simulink model "multiModePlanner"  (R2020b)
settings: Solver=FixedStepAuto  StartTime=0.0  StopTime=inf  FixedStep=0.5  MinStep=0.1  RelTol=1e-3
undefined symbols (not defined in the file or in its folder): DiscIntNeverNeededParam
settings Model: Creator=Ron  LastModifiedBy=cosorio
settings DataIOCC: ReturnWorkspaceOutputs=off

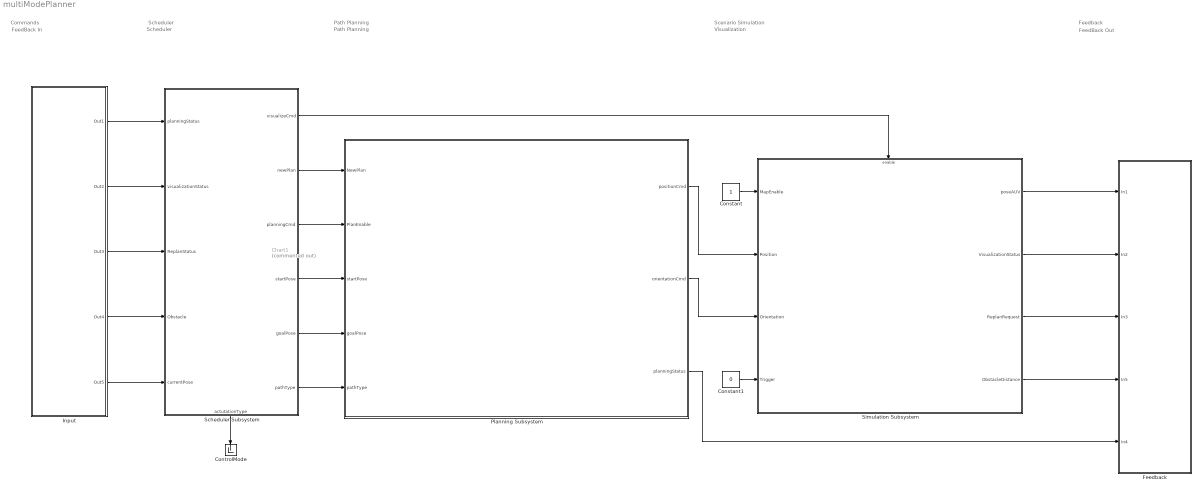
== system multiModePlanner ==
  note: Path Planning
  note: FeedBack In
  note: FeedBack Out
  note: Scheduler
  note: Path Planning
  note: Visualization
  note: Scheduler
  note: Commands
  note: Feedback
  note: Scenario Simulation
  " Feedback  " : Subsystem
  Chart1 : Stateflow chart  Commented=on  TreatAsAtomicUnit=on
  Constant : Constant
  Constant1 : Constant  Value=0
  ControlMode : Terminator
  Input : Subsystem
  Planning Subsystem : Subsystem
  Scheduler Subsystem : Stateflow chart  TreatAsAtomicUnit=on
      settings: PortSchema="{\"entries\":[{\"content\":{\"sides\":[{\"content\":{\"connectorIds\":[\"In1\",\"In2\",\"In3\",\"In4\",\"In5\"]},\"type\":\"ConnectorPlacement.EquallySpacedRectSide\",\"uuid\":\"1bd6ddfe-5f8a-4931-8a8b-c6c0dc399580\"},{\"content\":{\"connectorIds\":[\"Out5\",\"Out6\",\"Out1\",\"Out2\",\"Out3\",\"Out4\"],\"side\":\"RIGHT\"},\"type\":\"ConnectorPlacement.EquallySpacedRectSide\",\"uuid\":\"6c4632f4-be38-4d28-9a15-6462af5cd566\"},{\"content\":{\"connectorIds\":[],\"side\":\"TOP\"},\"type\":\"ConnectorPlacement.EquallySpacedRectSide\",\"uuid\":\"b3d6ad09-cf01-4725-a10c-99a606f09fed\"},{\"content\":{\"connectorIds\":[\"Out7\"],\"side\":\"BOTTOM\"},\"type\":\"ConnectorPlacement.EquallySpacedRectSide\",\"uuid\":\"99f6d769-50a8-4e4e-9c90-fdb41bcec8c1\"}]},\"type\":\"ConnectorPlacement.EquallySpacedConnector\",\"uuid\":\"51f2bfa3-614b-4c29-a9f7-1bf781273fcd\"}],\"packageUris\":[\"http://schema.mathworks.com/mf0/Connector/19700101\"],\"version\":\"1.0\"}"
  Simulation Subsystem : Subsystem
  wires:
  Constant/1 -> Simulation Subsystem/1(MapEnable)
  Constant1/1 -> Simulation Subsystem/4(Trigger)
  Scheduler Subsystem/5(visualizeCmd) -> Simulation Subsystem/Enable
  Scheduler Subsystem/7(actutationType) -> ControlMode/1
  Scheduler Subsystem/6(newPlan) -> Planning Subsystem/1(NewPlan)
  Scheduler Subsystem/1(planningCmd) -> Planning Subsystem/2(" PlanEnable")
  Scheduler Subsystem/2(startPose) -> Planning Subsystem/3(startPose)
  Scheduler Subsystem/3(goalPose) -> Planning Subsystem/4(goalPose)
  Scheduler Subsystem/4(pathType) -> Planning Subsystem/5(pathType)
  Planning Subsystem/1(positionCmd) -> Simulation Subsystem/2(Position)
  Planning Subsystem/2(orientationCmd) -> Simulation Subsystem/3(Orientation)
  Input/1(Out1) -> Scheduler Subsystem/1(planningStatus)
  Input/2(Out2) -> Scheduler Subsystem/2(visualizationStatus)
  Input/3(Out3) -> Scheduler Subsystem/3(ReplanStatus)
  Input/4(Out4) -> Scheduler Subsystem/4(Obstacle)
  Input/5(Out5) -> Scheduler Subsystem/5(currentPose)
  Simulation Subsystem/1(poseAUV) -> " Feedback  "/1(In1)
  Simulation Subsystem/2(VisualizationStatus) -> " Feedback  "/2(In2)
  Simulation Subsystem/3(ReplanRequest) -> " Feedback  "/3(In3)
  Planning Subsystem/3(planningStatus) -> " Feedback  "/5(In4)
  Simulation Subsystem/4(ObstacleDistance) -> " Feedback  "/4(In5)

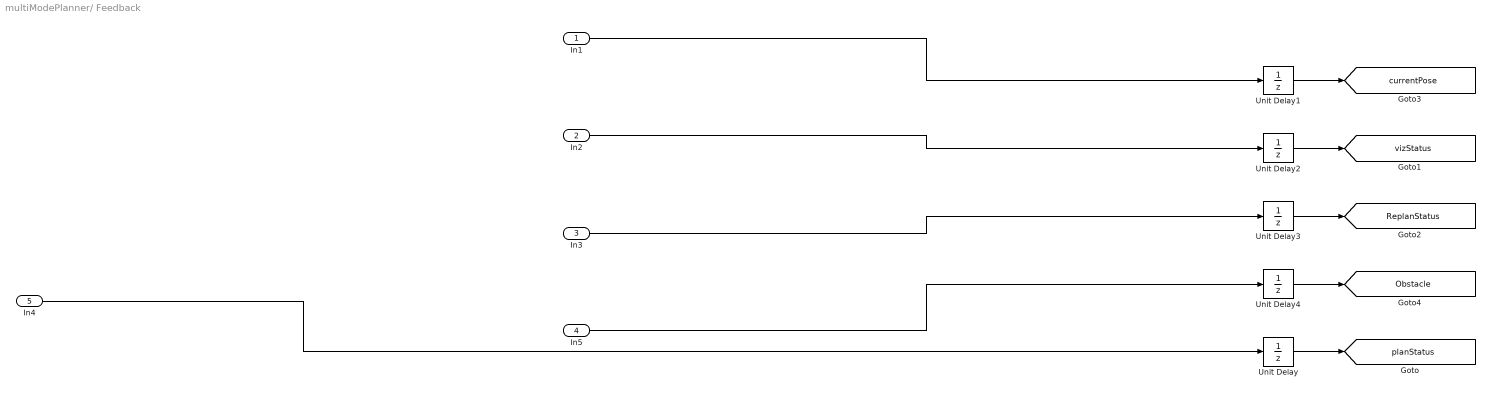
== system multiModePlanner/ Feedback   ==
  In1 : Inport
  In2 : Inport  Port=2
  In3 : Inport  Port=3
  In5 : Inport  Port=4
  In4 : Inport  Port=5
  Unit Delay{,1..3} (4 alike) : UnitDelay  SampleTime=-1  HasFrameUpgradeWarning=on
  Unit Delay4 : UnitDelay  InitialCondition=[0]  SampleTime=-1  HasFrameUpgradeWarning=on
  tag scope: Obstacle=global, ReplanStatus=global, currentPose=global, planStatus=global, vizStatus=global
  wires:
  Unit Delay3/1 -> [ReplanStatus]
  In2/1 -> Unit Delay2/1
  Unit Delay1/1 -> [currentPose]
  Unit Delay/1 -> [planStatus]
  In3/1 -> Unit Delay3/1
  Unit Delay4/1 -> [Obstacle]
  Unit Delay2/1 -> [vizStatus]
  In1/1 -> Unit Delay1/1
  In5/1 -> Unit Delay4/1
  In4/1 -> Unit Delay/1

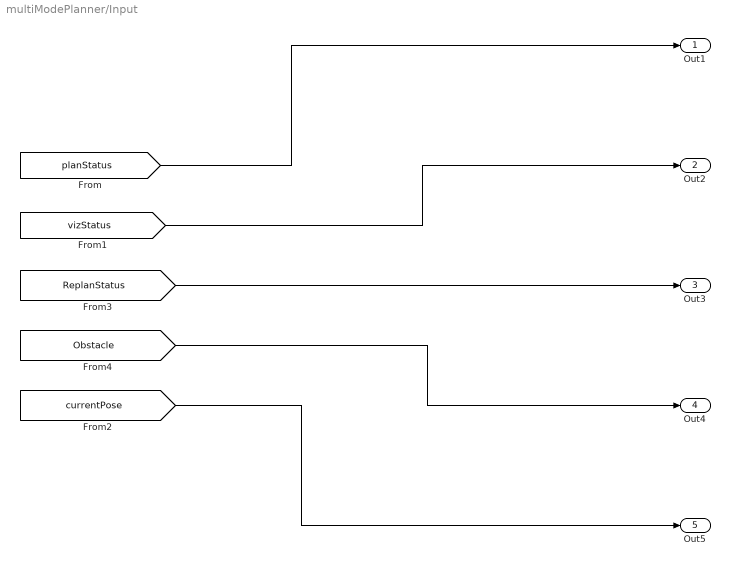
== system multiModePlanner/Input ==
  Out1 : Outport
  Out2 : Outport  Port=2
  Out3 : Outport  Port=3
  Out4 : Outport  Port=4
  Out5 : Outport  Port=5
  wires:
  [vizStatus] -> Out2/1
  [ReplanStatus] -> Out3/1
  [planStatus] -> Out1/1
  [currentPose] -> Out5/1
  [Obstacle] -> Out4/1

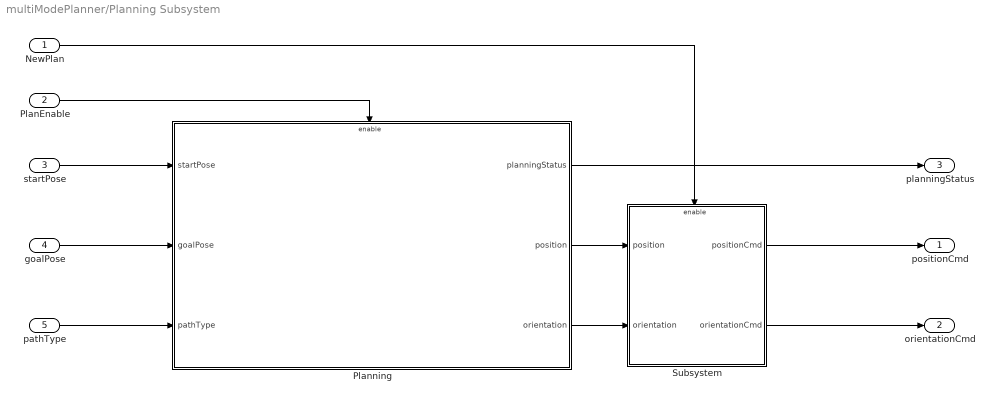
== system multiModePlanner/Planning Subsystem ==
  NewPlan : Inport
  " PlanEnable" : Inport  Port=2
  startPose : Inport  Port=3
  goalPose : Inport  Port=4
  pathType : Inport  Port=5
  Planning : Subsystem
  Subsystem : Subsystem
  positionCmd : Outport
  orientationCmd : Outport  Port=2
  planningStatus : Outport  Port=3
  wires:
  Planning/1(planningStatus) -> planningStatus/1
  Planning/3(orientation) -> Subsystem/2(orientation)
  pathType/1 -> Planning/3(pathType)
  Planning/2(position) -> Subsystem/1(position)
  Subsystem/1(positionCmd) -> positionCmd/1
  startPose/1 -> Planning/1(startPose)
  Subsystem/2(orientationCmd) -> orientationCmd/1
  " PlanEnable"/1 -> Planning/Enable
  goalPose/1 -> Planning/2(goalPose)
  NewPlan/1 -> Subsystem/Enable

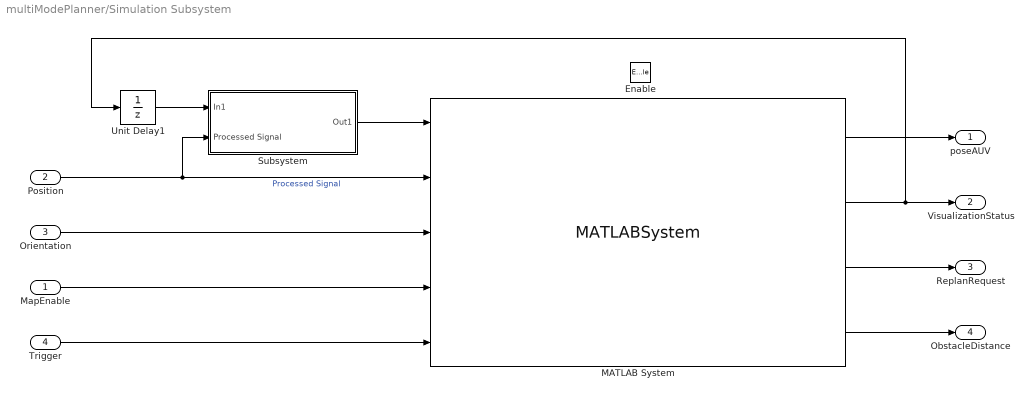
== system multiModePlanner/Simulation Subsystem ==
  MapEnable : Inport
  Position : Inport  Port=2
  Orientation : Inport  Port=3
  Trigger : Inport  Port=4
  Enable : EnablePort  PropagateVarSize=During execution
  MATLAB System : MATLABSystem  System=auvScenarioHillsSimulation_MultiMode  RollAccuracy=0.2  PitchAccuracy=0.2  YawAccuracy=0.2  PositionAccuracy=1  VelocityAccuracy=0.05
      mask Type: auvScenarioHillsSimulation_MultiMode
      mask Display:
      | disp('auvScenarioHillsSimulation_MultiMode');
      | port_label('input',1,'counter');
      | port_label('input',2,'position');
      | port_label('input',3,'orientation');
      | port_label('input',4,'mapEnable');
      | port_label('input',5,'trigger');
      | port_label('output',1,'poseUUV');
      | port_label('output',2,'VisualizationStatus');
      | port_label('output',3,'ReplanRequest');
      | port_label('output',4,'Obstacle');
  Subsystem : Subsystem
  Unit Delay1 : UnitDelay  SampleTime=-1  HasFrameUpgradeWarning=on
  poseAUV : Outport
  VisualizationStatus : Outport  Port=2
  ReplanRequest : Outport  Port=3
  ObstacleDistance : Outport  Port=4
  wires:
  Orientation/1 -> MATLAB System/3
  Trigger/1 -> MATLAB System/5
  MapEnable/1 -> MATLAB System/4
  MATLAB System/1 -> poseAUV/1
  MATLAB System/2 -> Unit Delay1/1, VisualizationStatus/1
  MATLAB System/3 -> ReplanRequest/1
  MATLAB System/4 -> ObstacleDistance/1
  Position/1 -> Subsystem/2(Processed Signal), MATLAB System/2  "Processed Signal"
  Unit Delay1/1 -> Subsystem/1(In1)
  Subsystem/1(Out1) -> MATLAB System/1

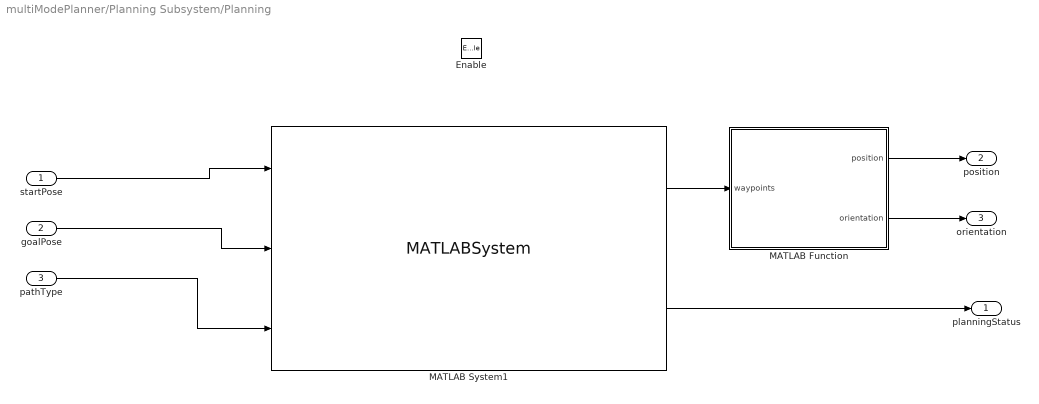
== system multiModePlanner/Planning Subsystem/Planning ==
  startPose : Inport
  goalPose : Inport  Port=2
  pathType : Inport  Port=3
  Enable : EnablePort  PropagateVarSize=During execution
  MATLAB Function : MATLAB Function  TreatAsAtomicUnit=on
  MATLAB System1 : MATLABSystem  System=auvPathPlanner_MultiMode  occMap=UUVSceneLowResMap3.mat  maxRollAngle=pi/6  airSpeed=8  flightPathAngleLimit=[ -0.1, 0.1 ]  bounds=[ -250, 250; -250, 250; -250, 250; -pi, pi ]  searchCoordinates=[ 400, 400 ]  searchFOV=10  bouyPostions=[ -150, 150, -150, -150, 150, 0 ]  bouyCoverage=300  SimulateUsing=Interpreted execution
      mask Type: auvPathPlanner_MultiMode
      mask Display:
      | disp('auvPathPlanner_MultiMode');
      | port_label('input',1,'startPose');
      | port_label('input',2,'goalPose');
      | port_label('input',3,'pathType');
      | port_label('output',1,'waypoints');
      | port_label('output',2,'planningStatus');
  planningStatus : Outport
  position : Outport  Port=2
  orientation : Outport  Port=3
  wires:
  MATLAB System1/1 -> MATLAB Function/1(waypoints)
  pathType/1 -> MATLAB System1/3
  goalPose/1 -> MATLAB System1/2
  MATLAB System1/2 -> planningStatus/1
  startPose/1 -> MATLAB System1/1
  MATLAB Function/1(position) -> position/1
  MATLAB Function/2(orientation) -> orientation/1

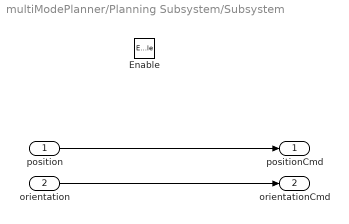
== system multiModePlanner/Planning Subsystem/Subsystem ==
  position : Inport
  orientation : Inport  Port=2
  Enable : EnablePort
  positionCmd : Outport
  orientationCmd : Outport  Port=2
  wires:
  position/1 -> positionCmd/1
  orientation/1 -> orientationCmd/1

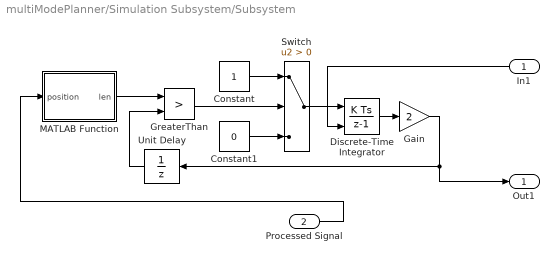
== system multiModePlanner/Simulation Subsystem/Subsystem ==
  In1 : Inport
  Processed Signal : Inport  Port=2
  Constant : Constant
  Constant1 : Constant  Value=0
  Discrete-Time Integrator : DiscreteIntegrator  ExternalReset=rising  SampleTime=-1  ICPrevOutput=DiscIntNeverNeededParam  ICPrevScaledInput=DiscIntNeverNeededParam
  Gain : Gain  Gain=2
  GreaterThan : RelationalOperator  Operator=>  OutDataTypeStr=boolean  RndMeth=Simplest
  MATLAB Function : MATLAB Function  TreatAsAtomicUnit=on
  Switch : Switch  Criteria=u2 > Threshold
  Unit Delay : UnitDelay  SampleTime=-1  HasFrameUpgradeWarning=on
  Out1 : Outport
  wires:
  Processed Signal/1 -> MATLAB Function/1(position)
  GreaterThan/1 -> Switch/2
  Switch/1 -> Discrete-Time Integrator/1
  Constant1/1 -> Switch/3
  Unit Delay/1 -> GreaterThan/2
  Constant/1 -> Switch/1
  MATLAB Function/1(len) -> GreaterThan/1
  Discrete-Time Integrator/1 -> Gain/1
  Gain/1 -> Out1/1, Unit Delay/1
  In1/1 -> Discrete-Time Integrator/2

== stateflow chart multiModePlanner/Chart1 ==
  state Dive
  state Simulation
    state Dive
    state Survey
    state Search
    state Inspect
    state Resurface
    (default) -> Simulation.Dive
    Simulation -> Simulation.Dive [order 4] : startDive
    Simulation.Survey -> Simulation [order 2] : diveCompleted
    Simulation -> Simulation.Survey [order 3] : startSurvey
    Simulation.Survey -> Simulation [order 1] : blackBoxNotDetected
    Simulation.Search -> Simulation : blackBoxDetected
    Simulation -> Simulation.Search [order 2] : startSearch
    Simulation.Inspect -> Simulation : obstacleDetected
    Simulation -> Simulation.Inspect [order 1] : startInspection
    Simulation -> Simulation.Resurface [order 5] : startResurface
    Simulation.Resurface -> Simulation : blackBoxDetected
  state Survey
  state Search
  state Inspect
  state Resurface
  (default) -> Dive
  Dive -> Simulation [order 1] : startDive
  Dive -> Resurface [order 2] : faultDetected
  Simulation -> Survey [order 4] : diveCompleted
  Survey -> Simulation [order 1] : startSurvey
  Simulation -> Survey [order 5] : blackBoxNotDetected
  Survey -> Resurface [order 2] : faultDetected
  Simulation -> Search [order 3] : blackBoxDetected
  Search -> Simulation [order 1] : startSearch
  Search -> Resurface [order 2] : faultDetected
  Simulation -> Inspect [order 2] : obstacleDetected
  Inspect -> Simulation [order 1] : startInspection
  Inspect -> Resurface [order 2] : faultDetected
  Simulation -> Resurface [order 1] : blackBoxLocated
  Resurface -> Simulation : startResurface

== matlab function multiModePlanner/Simulation Subsystem/Subsystem/MATLAB Function ==
  data: position input size=[20000 3]; len output
function len = fcn(position)

len= length(position);

end

== matlab function multiModePlanner/Planning Subsystem/Planning/MATLAB Function ==
  data: waypoints input size=[20000 7]; position output size=[20000 3]; orientation output size=[20000 3]
function [position,orientation] = convertWaypoints(waypoints)
coder.extrinsic('plot3','load'); 

% figure
% plot3(waypoints(:,1),...
%     waypoints(:,2), ...
%     waypoints(:,3), "LineWidth",2,"Color","r");

position = waypoints(:,1:3);

% if (size(waypoints,2)==4)
%orientation = [waypoints(:,4) zeros(939,1) zeros(939,1)];
% else
 orientation = [waypoints(:,4) zeros(length(waypoints(:,4)),1) zeros(length(waypoints(:,4)),1)];
% end

== stateflow chart multiModePlanner/Scheduler Subsystem ==
  state Dive
    en:
    newPlan = 1;
    actutationType = 1;
    planningCmd = 1;
    visualizeCmd = 0;
    startPose = [-150,-150,150,0];
    goalPose = [-150,-150,80,0];
    pathType = 3;
  state Visuallize1
    en:
    newPlan = 0;
    planningCmd = 0;
    visualizeCmd = 1;
  state Search
    en:
    newPlan = 1;
    planningCmd = 1;
    visualizeCmd = 0;
    startPose =  [-150,-150,80,0];
    goalPose =[0,0,0,0]
    pathType = 1;
  state Visuallize2
    en:
    newPlan = 0;
    planningCmd = 0;
    visualizeCmd = 1;
  state Survey
    en:
    newPlan = 1;
    planningCmd = 1;
    visualizeCmd = 0;
    startPose =[-17,20,50,0];
    goalPose =[-17,20,20,0]
    pathType = 3;
  state Visuallize3
    en:
    newPlan = 0;
    planningCmd = 0;
    visualizeCmd = 1;
  state Inspect
    en:
    planningCmd = 1;
    startPose = Obstacle(1,2:5)
    goalPose =[-17,20,20,0];
    pathType = 2;
    du:
    planningCmd = 0;
  state Visuallize4
    en:
    newPlan = 1;
    planningCmd = 0;
    visualizeCmd = 1;
    actutationType = 2;
  (default) -> Dive
  Dive -> Visuallize1 : [planningStatus==1]
  Visuallize1 -> Search : [visualizationStatus ==1]
  Search -> Visuallize2 : [planningStatus==1]
  Visuallize2 -> Survey : [visualizationStatus ==1]
  Survey -> Visuallize3 : [planningStatus==1]
  Visuallize3 -> Inspect : [ReplanStatus == 1]
  Inspect -> Visuallize4 : [planningStatus==1 && isequal(currentPose,startPose)]
  Visuallize4 -> (junction 58) : [visualizationStatus ==1]
  (junction 58) -> (junction 61)
  data: planningCmd output; startPose output; goalPose output; pathType output; visualizeCmd output; planningStatus input size=[1 1]; visualizationStatus input; ReplanStatus input; Obstacle input; newPlan output; actutationType output; currentPose input
